simulink subsystem "CasADi_freetf"  (R2025a)
settings: Solver=VariableStepAuto  StartTime=0.0  StopTime=10.0  RelTol=1e-3
settings Model: Creator=thatf  LastModifiedBy=thatf

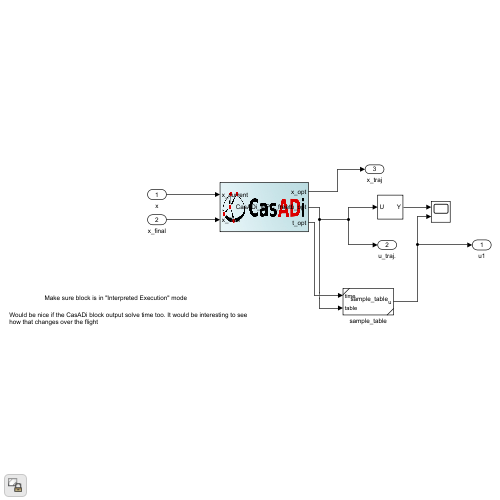
[thumbnail: Simulink's stored preview of the top-level diagram]
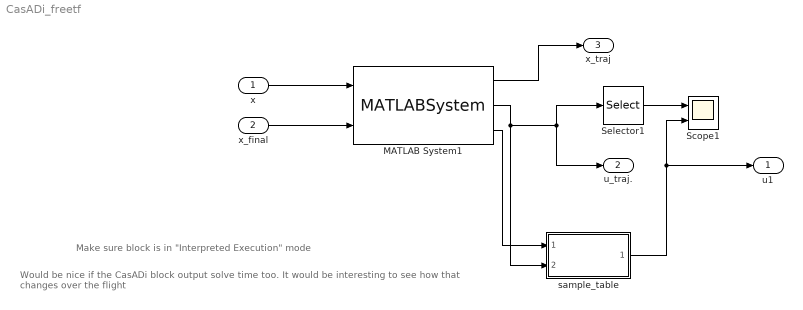
== system CasADi_freetf ==
  note: Make sure block is in "Interpreted Execution" mode
  note: Would be nice if the CasADi block output solve time too. It would be interesting to see how that changes over the flight
  x : Inport
  x_final : Inport  Port=2
  MATLAB System1 : MATLABSystem  System=CasADi_MPC_freetf  vehicle=vehicle  steps=steps  max_iter=400  x_initial=x0  SimulateUsing=Interpreted execution  max_t_step=0.5  x_final=xf
      mask Type: CasADi_MPC_freetf
  Scope1 : Scope  NumInputPorts=2
      settings: ActiveDisplayYMinimum=-0.05785  ActiveDisplayYMaximum=0.52066  DataLoggingVariableName=ScopeData3
  Selector1 : Selector  NumberOfDimensions=2  InputPortWidth=3  IndexOptions=Index vector (dialog),Select all  Indices=[1],1  OutputSizes=1,1
  sample_table : Subsystem  ReferencedSubsystem=sample_table
  u1 : Outport
  u_traj. : Outport  Port=2
  x_traj : Outport  Port=3
  wires:
  x/1 -> MATLAB System1/1
  MATLAB System1/1 -> x_traj/1
  MATLAB System1/2 -> u_traj./1, Selector1/1, sample_table/2
  x_final/1 -> MATLAB System1/2
  Selector1/1 -> Scope1/1
  sample_table/1 -> Scope1/2, u1/1
  MATLAB System1/3 -> sample_table/1
